simulink model "Hw5PID"  (R2023b)
settings: Solver=VariableStepAuto  StartTime=0.0  StopTime=10.0  RelTol=1e-3
libraries: simulink_extras x1
settings Model: Creator=Owner  LastModifiedBy=Owner

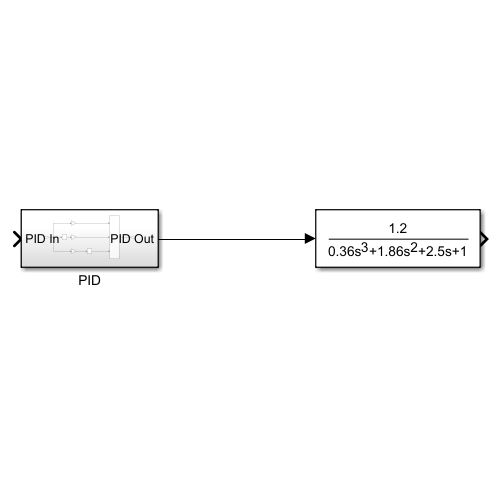
[thumbnail: Simulink's stored preview of the top-level diagram]
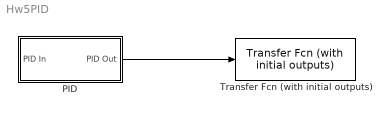
== system Hw5PID ==
  PID : Subsystem
  Transfer Fcn (with initial outputs) : simulink_extras/Additional Linear/Transfer Fcn (with initial outputs)  N=[1.2]  D=[0.36 1.86 2.5 1]  Y0=.5  U0=0
  wires:
  PID/1(PID Out) -> Transfer Fcn (with initial outputs)/1

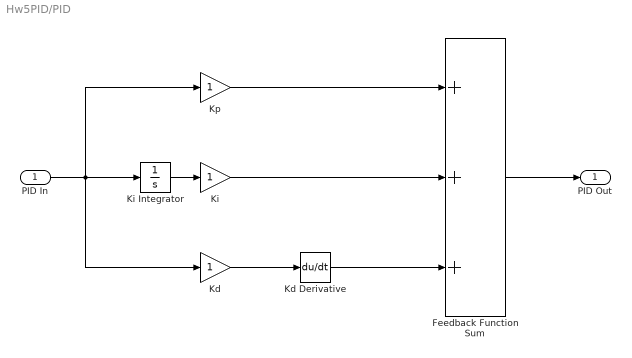
== system Hw5PID/PID ==
  PID In : Inport
  Feedback Function Sum : Sum  Inputs=+++
  Kd : Gain
  Kd Derivative : Derivative
  Ki : Gain
  Ki Integrator : Integrator
  Kp : Gain
  PID Out : Outport
  wires:
  PID In/1 -> Kd/1, Kp/1, Ki Integrator/1
  Kd/1 -> Kd Derivative/1
  Ki Integrator/1 -> Ki/1
  Kd Derivative/1 -> Feedback Function Sum/3
  Kp/1 -> Feedback Function Sum/1
  Ki/1 -> Feedback Function Sum/2
  Feedback Function Sum/1 -> PID Out/1
